simulink model "simlink"  (R2022b)
settings: Solver=VariableStepAuto  StartTime=0.0  StopTime=0  RelTol=1e-3
libraries: visionsources x1
settings Model: Creator=ECAD -24  LastModifiedBy=ECAD -24

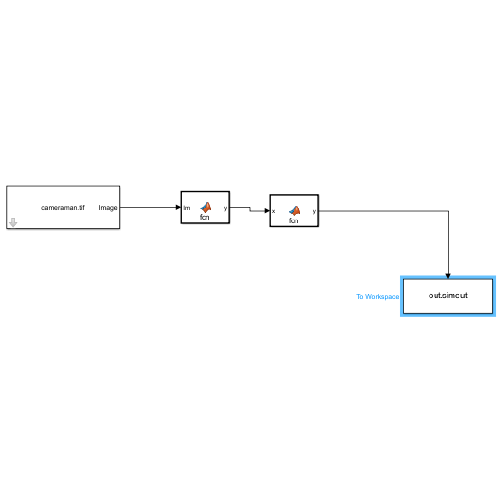
[thumbnail: Simulink's stored preview of the top-level diagram]
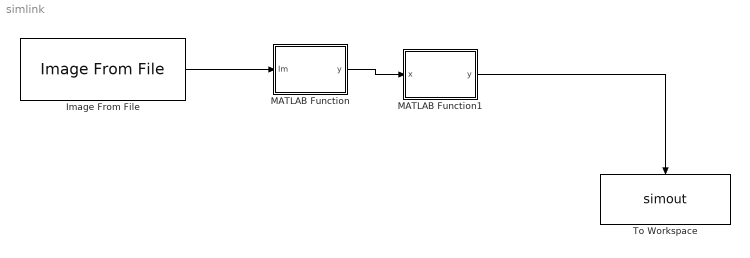
== system simlink ==
  Image From File : visionsources/Image From File  Tag=vipblks_nd  FileName=C:\Users\ECAD -24\Desktop\21ucc125_lab6\cameraman.tif  Ts=inf  imagePorts=One multidimensional signal  OutPortLabels=R|G|B  ImageDataType=Inherit from input image  sdImageDataType=uint(8)  Signed=on  WordLength=16  FractionLengthMode=User-defined  FractionLength=15
  MATLAB Function : MATLAB Function  TreatAsAtomicUnit=on
  MATLAB Function1 : MATLAB Function  TreatAsAtomicUnit=on
  To Workspace : ToWorkspace  VariableName=simout  SampleTime=-1
      settings: Save2DSignal=2-D array (concatenate along first dimension)
  wires:
  Image From File/1 -> MATLAB Function/1(Im)
  MATLAB Function/1(y) -> MATLAB Function1/1(x)
  MATLAB Function1/1(y) -> To Workspace/1

== matlab function simlink/MATLAB Function ==
  data: Im input; y output
function y = fcn(Im)
coder.extrinsic('dct2')
dct_coeff = dct2(Im);
M=256;
N=256;
z = zeros(M,N);
for i = 1:M
    for j = 1: N
        if(i<=M/2 && j<=N/2)
            z(i,j) = dct_coeff(i,j);
        else
            z(i,j) = z(i,j);
        end
    end
end
y =z;

== matlab function simlink/MATLAB Function1 ==
  data: x input; y output
function y = fcn(x)
[M,N] = size(x);
coder.extrinsic('idct2');
zout = zeros(M,N);
zout = idct(x);

y = zout;
